simulink model "stateflow_template"  (R2018b)
settings: Solver=FixedStepDiscrete  StartTime=0.0  StopTime=10.0  FixedStep=1  RelTol=1e-3
settings Model: Creator=cris  LastModifiedBy=cris

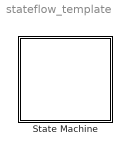
== system stateflow_template ==
  State Machine : Stateflow chart  TreatAsAtomicUnit=on

== stateflow chart stateflow_template/State Machine ==
